simulink subsystem "Power_limitation_old"  (R2022a)
settings: Solver=VariableStepAuto  StartTime=0.0  StopTime=10.0  RelTol=1e-3
settings Model: Creator=jutri  LastModifiedBy=Usuario
settings ModelReferenceCC: EnableRefExpFcnMdlSchedulingChecks=off
settings RTWCC: Description=Generic Real-Time Target  GPUComputeCapability=5.0

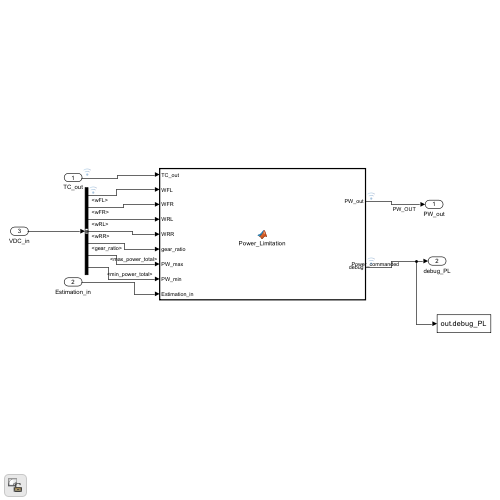
[thumbnail: Simulink's stored preview of the top-level diagram]
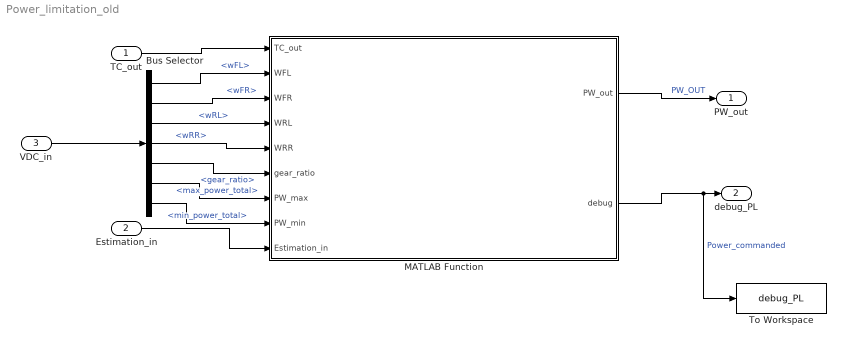
== system Power_limitation_old ==
  TC_out : Inport
  Estimation_in : Inport  Port=2
  VDC_in : Inport  Port=3
  Bus Selector : BusSelector  OutputSignals=sensors_in.encoder.wFL,sensors_in.encoder.wFR,sensors_in.encoder.wRL,sensors_in.encoder.wRR,param.gear_ratio,param.max_power_total,param.min_power_total
  MATLAB Function : MATLAB Function  TreatAsAtomicUnit=on
  To Workspace : ToWorkspace  VariableName=debug_PL  SaveFormat=Timeseries  SampleTime=-1
  PW_out : Outport
  debug_PL : Outport  Port=2
  wires:
  Estimation_in/1 -> MATLAB Function/9(Estimation_in)
  TC_out/1 -> MATLAB Function/1(TC_out)
  MATLAB Function/2(debug) -> debug_PL/1, To Workspace/1  "Power_commanded"
  MATLAB Function/1(PW_out) -> PW_out/1  "PW_OUT"
  VDC_in/1 -> Bus Selector/1
  Bus Selector/3 -> MATLAB Function/4(WRL)  "<wRL>"
  Bus Selector/4 -> MATLAB Function/5(WRR)  "<wRR>"
  Bus Selector/5 -> MATLAB Function/6(gear_ratio)  "<gear_ratio>"
  Bus Selector/6 -> MATLAB Function/7(PW_max)  "<max_power_total>"
  Bus Selector/2 -> MATLAB Function/3(WFR)  "<wFR>"
  Bus Selector/1 -> MATLAB Function/2(WFL)  "<wFL>"
  Bus Selector/7 -> MATLAB Function/8(PW_min)  "<min_power_total>"

== matlab function Power_limitation_old/MATLAB Function ==
  data: TC_out input; WFL input; WFR input; WRL input; WRR input; PW_out output; gear_ratio input; PW_max input; debug output; PW_min input; Estimation_in input
function [PW_out, debug] = Power_Limitation(TC_out, WFL, WFR, WRL, WRR, gear_ratio, PW_max, PW_min, Estimation_in)

MS = [WFR; WFL; WRR; WRL] .* gear_ratio;
PW = TC_out .* MS;
PW_total = sum(PW);

if (PW_total > PW_max)
    PW_extra = (PW_total-PW_max)/PW_total;
    for i=1:4                                        %Para hacerlo 2wd (cuando sea 2wd la simulación) solo hay que cambiar este a i=3:4 y el que comprueba potencia mínima
        TC_out(i) = TC_out(i) * (1-PW_extra);
    end
elseif (PW_total < PW_min)
    PW_extra = (PW_total - PW_min)/PW_total;
    for i=1:4
        TC_out(i) = TC_out(i) * (1-PW_extra);
    end
end

PW_out = TC_out;

debug = sum(PW_out .* MS);
